simulink model "AMR_gnss2udp_decoder_24a"  (R2024a)
settings: configuration reference "SharedConfig" (kept outside this file)
undefined symbols (not defined in the file): max_gnss_height, min_gnss_height, min_SVs2RTK, tstep
libraries: slrealtimeutilitieslib x7, simulink x2
settings Model: DataDictionary=configuration_dictionary.sldd  Creator=matlab.cut  LastModifiedBy=matlab.cut
settings ConfigSetRef: SourceName=SharedConfig

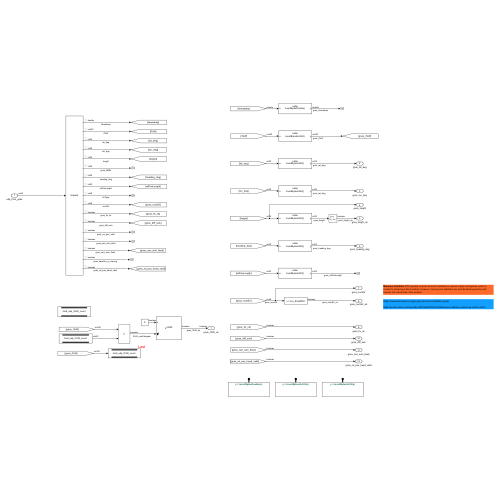
[thumbnail: Simulink's stored preview of the top-level diagram]
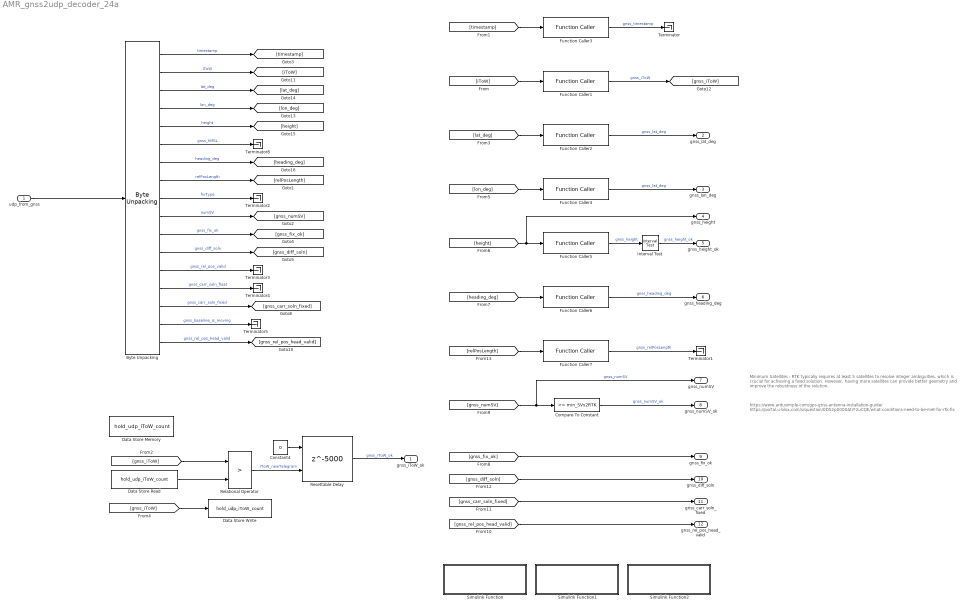
== system AMR_gnss2udp_decoder_24a ==
  note: https://www.ardusimple.com/gps-gnss-antenna-installation-guide/
      |
      | https://portal.u-blox.com/s/question/0D52p0000AtrF2uCQE/what-conditions-need-to-be-met-for-rtk-fix
  note: Minimum Satellites : RTK typically requires at least 5 satellites to resolve integer ambiguities, which is crucial for achieving a fixed solution. However, having more satellites can provide better geometry and improve the robustness of the solution.
  udp_from_gnss : Inport  OutDataTypeStr=uint8  PortDimensions=45
  Byte Unpacking : slrealtimeutilitieslib/Byte Unpacking  MaskUnpackedDataTypes={'double','uint32','int32','int32','int32','int32','int32','int32','uint8','uint8','boolean','boolean','boolean','boolean','boolean','boolean','boolean'}  MaskUnpackedDataSizes={1,1,1,1,1,1,1,1,1,1,1,1,1,1,1,1,1}  MaskAlignment=1
  Compare To Constant : simulink/Logic and Bit Operations/Compare To Constant  relop=>=  const=min_SVs2RTK  OutDataTypeStr=boolean
  Constant4 : Constant  Value=0  OutDataTypeStr=boolean
  Data Store Memory : DataStoreMemory  DataStoreName=hold_udp_iToW_count  WriteAfterWriteMsg=warning  ShowAdditionalParam=off  OutDataTypeStr=uint32  Dimensions=1
      settings: LockScale=on
  Data Store Read : DataStoreRead  DataStoreName=hold_udp_iToW_count  DataStoreElements=hold_udp_iToW_count  IndexOptions=Index vector (dialog)  Indices=1  OutputSizes=1
  Data Store Write : DataStoreWrite  ExecutionOrder=Last  DataStoreName=hold_udp_iToW_count  DataStoreElements=hold_udp_iToW_count  IndexOptions=Index vector (dialog)  Indices=1  OutputSizes=1
  Function Caller1 : FunctionCaller  FunctionPrototype=y = invertBytesUint32(u)  InputArgumentSpecifications=<Enter example>  OutputArgumentSpecifications=<Enter example>
  Function Caller{2,4..7} (5 alike) : FunctionCaller  FunctionPrototype=y = invertBytesInt32(u)  InputArgumentSpecifications=<Enter example>  OutputArgumentSpecifications=<Enter example>
  Function Caller3 : FunctionCaller  FunctionPrototype=y = invertBytesDouble(u)  InputArgumentSpecifications=<Enter example>  OutputArgumentSpecifications=<Enter example>
  Interval Test : simulink/Logic and Bit Operations/Interval Test  IntervalClosedRight=off  uplimit=min_gnss_height  IntervalClosedLeft=off  lowlimit=max_gnss_height  OutDataTypeStr=boolean
  Relational Operator : RelationalOperator  Operator=>  OutDataTypeStr=boolean  RndMeth=Simplest  InputSameDT=off
  Resettable Delay : Delay  DelayLength=5000  InitialCondition=1  ExternalReset=Rising  SampleTime=tstep
      settings: InputPortMap=u0,r5
  Simulink Function : Subsystem  TreatAsAtomicUnit=on
  Simulink Function1 : Subsystem  TreatAsAtomicUnit=on
  Simulink Function2 : Subsystem  TreatAsAtomicUnit=on
  Terminator{,1..5,8} (7 alike) : Terminator
  gnss_iToW_ok : Outport  OutDataTypeStr=boolean
  gnss_lat_deg : Outport  Port=2
  gnss_lon_deg : Outport  Port=3
  gnss_height : Outport  Port=4
  gnss_height_ok : Outport  Port=5
  gnss_heading_deg : Outport  Port=6
  gnss_numSV : Outport  Port=7
  gnss_numSV_ok : Outport  Port=8
  gnss_fix_ok : Outport  Port=9
  gnss_diff_soln : Outport  Port=10
  gnss_carr_soln_fixed : Outport  Port=11
  gnss_rel_pos_head_valid : Outport  Port=12
  wires:
  Byte Unpacking/10 -> [gnss_numSV]  "numSV"
  Byte Unpacking/11 -> [gnss_fix_ok]  "gnss_fix_ok"
  Byte Unpacking/9 -> Terminator2/1  "fixType"
  Byte Unpacking/12 -> [gnss_diff_soln]  "gnss_diff_soln"
  Byte Unpacking/5 -> [height]  "height"
  Byte Unpacking/13 -> Terminator3/1  "gnss_rel_pos_valid"
  Byte Unpacking/8 -> [relPosLength]  "relPosLength"
  Byte Unpacking/7 -> [heading_deg]  "heading_deg"
  Byte Unpacking/2 -> [iToW]  "iToW"
  Byte Unpacking/6 -> Terminator8/1  "gnss_hMSL"
  Byte Unpacking/1 -> [timestamp]  "timestamp"
  Byte Unpacking/3 -> [lat_deg]  "lat_deg"
  Byte Unpacking/14 -> Terminator4/1  "gnss_carr_soln_float"
  Byte Unpacking/4 -> [lon_deg]  "lon_deg"
  Byte Unpacking/15 -> [gnss_carr_soln_fixed]  "gnss_carr_soln_fixed"
  Byte Unpacking/16 -> Terminator5/1  "gnss_baseline_is_moving"
  udp_from_gnss/1 -> Byte Unpacking/1
  Byte Unpacking/17 -> [gnss_rel_pos_head_valid]  "gnss_rel_pos_head_valid"
  Resettable Delay/1 -> gnss_iToW_ok/1  "gnss_iToW_ok"
  Constant4/1 -> Resettable Delay/1
  Relational Operator/1 -> Resettable Delay/2  "iToW_newTelegram"
  Data Store Read/1 -> Relational Operator/2
  [gnss_iToW] -> Relational Operator/1
  [timestamp] -> Function Caller3/1
  [iToW] -> Function Caller1/1
  Function Caller1/1 -> [gnss_iToW]  "gnss_iToW"
  [gnss_iToW] -> Data Store Write/1
  [lat_deg] -> Function Caller2/1
  [lon_deg] -> Function Caller4/1
  [height] -> gnss_height/1, Function Caller5/1
  [heading_deg] -> Function Caller6/1
  Function Caller3/1 -> Terminator/1  "gnss_timestamp"
  Function Caller5/1 -> Interval Test/1  "gnss_height"
  [gnss_diff_soln] -> gnss_diff_soln/1
  [relPosLength] -> Function Caller7/1
  Function Caller7/1 -> Terminator1/1  "gnss_relPosLength"
  [gnss_numSV] -> gnss_numSV/1, Compare To Constant/1  "gnss_numSV"
  Interval Test/1 -> gnss_height_ok/1  "gnss_height_ok"
  Compare To Constant/1 -> gnss_numSV_ok/1  "gnss_numSV_ok"
  [gnss_fix_ok] -> gnss_fix_ok/1
  [gnss_carr_soln_fixed] -> gnss_carr_soln_fixed/1
  [gnss_rel_pos_head_valid] -> gnss_rel_pos_head_valid/1
  Function Caller2/1 -> gnss_lat_deg/1  "gnss_lat_deg"
  Function Caller4/1 -> gnss_lon_deg/1  "gnss_lat_deg"
  Function Caller6/1 -> gnss_heading_deg/1  "gnss_heading_deg"

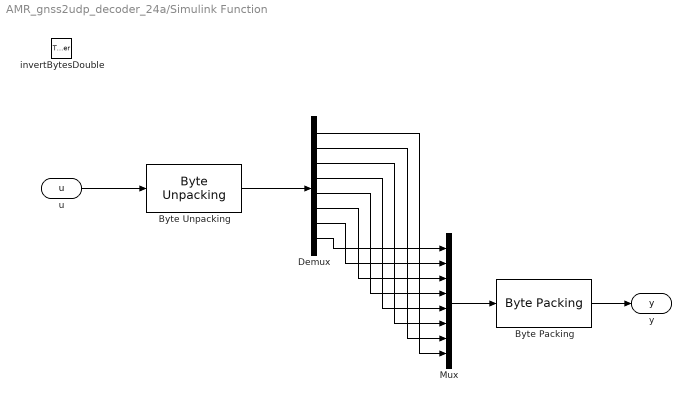
== system AMR_gnss2udp_decoder_24a/Simulink Function ==
  invertBytesDouble : TriggerPort  TriggerType=function-call  IsSimulinkFunction=on  FunctionName=invertBytesDouble  FunctionVisibility=scoped  VariantControl=(inherit)
  Byte Packing : slrealtimeutilitieslib/Byte Packing  MaskPackedDataType=double  MaskUnpackedDataTypes={['uint8']}  MaskAlignment=1
  Byte Unpacking : slrealtimeutilitieslib/Byte Unpacking  MaskUnpackedDataTypes={['uint8']}  MaskUnpackedDataSizes={[8]}  MaskAlignment=1
  Demux : Demux  Outputs=8
  Mux : Mux  Inputs=8
  u : ArgIn  DisableCoverage=on  ArgumentName=u
  y : ArgOut  DisableCoverage=on  ArgumentName=y
  wires:
  Byte Packing/1 -> y/1
  u/1 -> Byte Unpacking/1
  Mux/1 -> Byte Packing/1
  Demux/7 -> Mux/2
  Demux/6 -> Mux/3
  Demux/2 -> Mux/7
  Demux/1 -> Mux/8
  Demux/3 -> Mux/6
  Byte Unpacking/1 -> Demux/1
  Demux/8 -> Mux/1
  Demux/4 -> Mux/5
  Demux/5 -> Mux/4

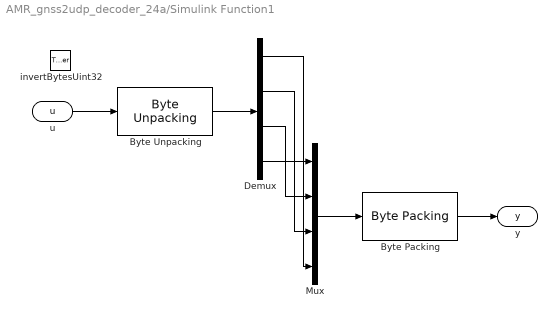
== system AMR_gnss2udp_decoder_24a/Simulink Function1 ==
  invertBytesUint32 : TriggerPort  TriggerType=function-call  IsSimulinkFunction=on  FunctionName=invertBytesUint32  FunctionVisibility=scoped  VariantControl=(inherit)
  Byte Packing : slrealtimeutilitieslib/Byte Packing  MaskPackedDataType=uint32  MaskUnpackedDataTypes={['uint8']}  MaskAlignment=1
  Byte Unpacking : slrealtimeutilitieslib/Byte Unpacking  MaskUnpackedDataTypes={['uint8']}  MaskUnpackedDataSizes={[4]}  MaskAlignment=1
  Demux : Demux
  Mux : Mux
  u : ArgIn  DisableCoverage=on  OutDataTypeStr=uint32  ArgumentName=u
  y : ArgOut  DisableCoverage=on  OutDataTypeStr=uint32  ArgumentName=y
  wires:
  Mux/1 -> Byte Packing/1
  u/1 -> Byte Unpacking/1
  Byte Unpacking/1 -> Demux/1
  Demux/4 -> Mux/1
  Demux/3 -> Mux/2
  Demux/2 -> Mux/3
  Demux/1 -> Mux/4
  Byte Packing/1 -> y/1

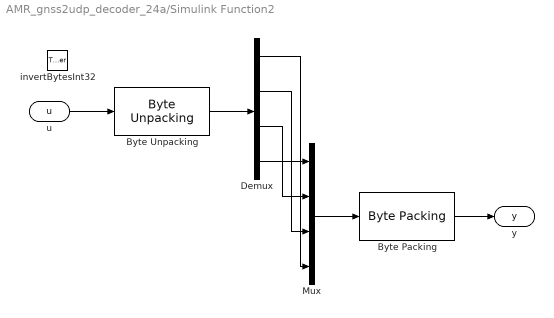
== system AMR_gnss2udp_decoder_24a/Simulink Function2 ==
  invertBytesInt32 : TriggerPort  TriggerType=function-call  IsSimulinkFunction=on  FunctionName=invertBytesInt32  FunctionVisibility=scoped  VariantControl=(inherit)
  Byte Packing : slrealtimeutilitieslib/Byte Packing  MaskPackedDataType=int32  MaskUnpackedDataTypes={['uint8']}  MaskAlignment=1
  Byte Unpacking : slrealtimeutilitieslib/Byte Unpacking  MaskUnpackedDataTypes={['uint8']}  MaskUnpackedDataSizes={[4]}  MaskAlignment=1
  Demux : Demux
  Mux : Mux
  u : ArgIn  DisableCoverage=on  OutDataTypeStr=int32  ArgumentName=u
  y : ArgOut  DisableCoverage=on  OutDataTypeStr=int32  ArgumentName=y
  wires:
  u/1 -> Byte Unpacking/1
  Mux/1 -> Byte Packing/1
  Demux/4 -> Mux/1
  Byte Packing/1 -> y/1
  Demux/1 -> Mux/4
  Demux/2 -> Mux/3
  Demux/3 -> Mux/2
  Byte Unpacking/1 -> Demux/1
